simulink model "boucle_fermee"  (R2018b)
settings: Solver=VariableStepAuto  StartTime=0.0  StopTime=1000  MaxStep=0.01  RelTol=1e-3
values from neighbouring files (symbols this model uses):
  alpha = 1+1/(2*k)    (= 2.75438596491)    [parametres_tp2.m]
  k = 0.285    [parametres_tp2.m]
settings Model: Creator=12003927  LastModifiedBy=12003927

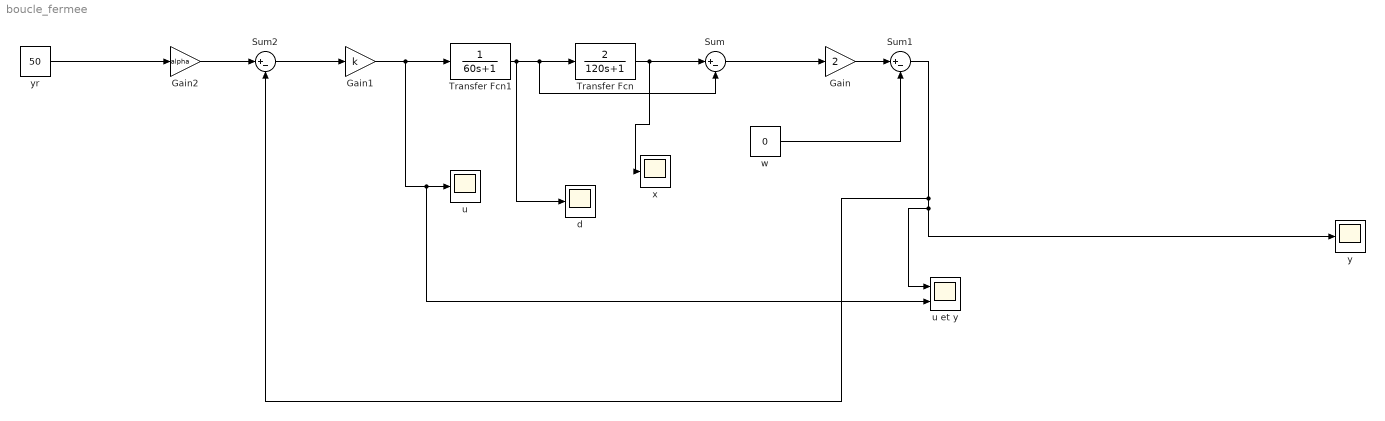
== system boucle_fermee ==
  Gain : Gain  Gain=2
  Gain1 : Gain  Gain=k
  Gain2 : Gain  Gain=alpha
  Sum : Sum  Inputs=|+-
  Sum1 : Sum  Inputs=|+-
  Sum2 : Sum  Inputs=|+-
  Transfer Fcn : TransferFcn  Numerator=2  Denominator=[120 1]
  Transfer Fcn1 : TransferFcn  Denominator=[60 1]
  d : Scope
  u : Scope
  u et y : Scope  NumInputPorts=2
  w : Constant  Value=0
  x : Scope
  y : Scope
  "yr " : Constant  Value=50
  wires:
  Transfer Fcn1/1 -> d/1, Sum/2, Transfer Fcn/1
  Sum/1 -> Gain/1
  Transfer Fcn/1 -> x/1, Sum/1
  w/1 -> Sum1/2
  Gain/1 -> Sum1/1
  Sum2/1 -> Gain1/1
  Sum1/1 -> Sum2/2, u et y/1, y/1
  Gain1/1 -> u et y/2, u/1, Transfer Fcn1/1
  Gain2/1 -> Sum2/1
  "yr "/1 -> Gain2/1
